simulink model "MPC(废稿)"  (R2023a)
settings: Solver=VariableStepAuto  StartTime=0.0  StopTime=50  RelTol=1e-3
settings Model: Creator=c  LastModifiedBy=c

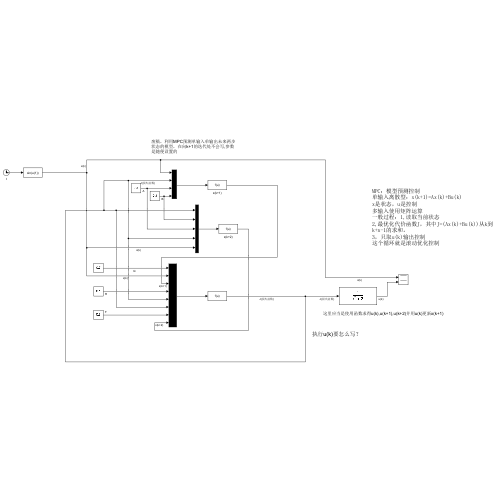
[thumbnail: Simulink's stored preview of the top-level diagram]
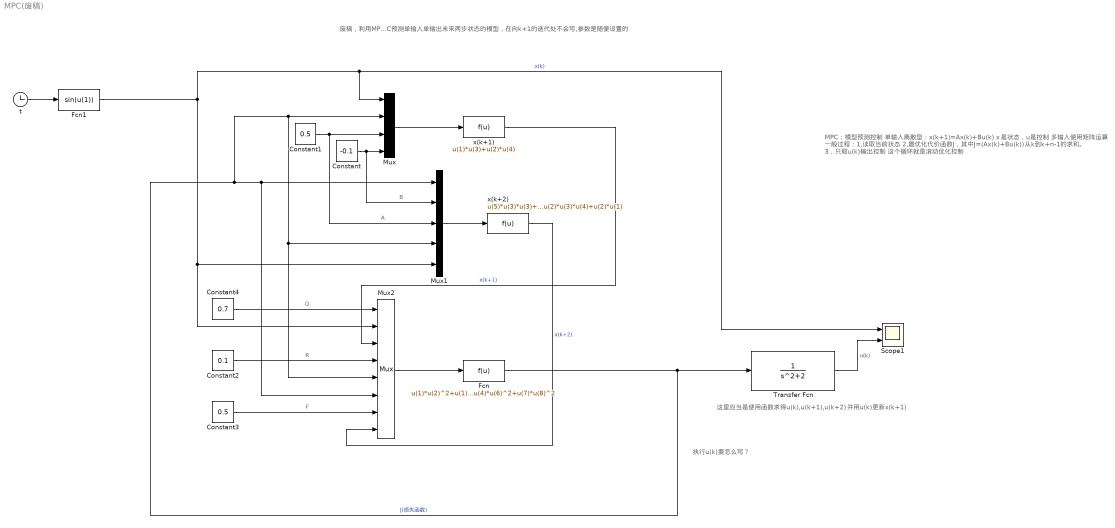
== system MPC(废稿) ==
  note: 废稿，利用MPC预测单输入单输出未来两步状态的模型，在向k+1的迭代处不会写,参数是随便设置的
  note: 这里应当是使用函数求得u(k),u(k+1),u(k+2)并用u(k)更新x(k+1)
  note: 执行u(k)要怎么写？
  note: MPC：模型预测控制
      | 单输入离散型：x(k+1)=Ax(k)+Bu(k)
      | x是状态，u是控制
      | 多输入使用矩阵运算
      | 一般过程：1,读取当前状态
      | 2,最优化代价函数J，其中J=(Ax(k)+Bu(k))从k到k+n-1的求和。
      | 3，只取u(k)输出控制
      | 这个循环就是滚动优化控制
  Constant : Constant  Value=-0.1
  Constant1 : Constant  Value=0.5
  Constant2 : Constant  Value=0.1
  Constant3 : Constant  Value=0.5
  Constant4 : Constant  Value=0.7
  Fcn : Fcn  Expr=u(1)*u(2)^2+u(1)*u(3)^2+u(4)*u(5)^2+u(4)*u(6)^2+u(7)*u(8)^2
  Fcn1 : Fcn  Expr=sin(u(1))
  Mux : Mux
  Mux1 : Mux  Inputs=5
  Mux2 : Mux  Inputs=8
  Scope1 : Scope  NumInputPorts=2
  Transfer Fcn : TransferFcn  Denominator=[1 0 2]
  t : Clock
  x(k+1) : Fcn  Expr=u(1)*u(3)+u(2)*u(4)
  x(k+2) : Fcn  Expr=u(5)*u(3)*u(3)+u(2)*u(3)*u(4)+u(2)*u(1)
  wires:
  Mux/1 -> x(k+1)/1
  Constant/1 -> Mux1/2, Mux/4  "B"
  Mux1/1 -> x(k+2)/1
  Constant1/1 -> Mux1/3, Mux/3  "A"
  Fcn/1 -> Transfer Fcn/1, Mux1/4, Mux2/5, Mux/2, Mux2/6, Mux1/1  "J(损失函数)"
  Mux2/1 -> Fcn/1
  Constant2/1 -> Mux2/4  "R"
  Constant3/1 -> Mux2/7  "F"
  x(k+2)/1 -> Mux2/8  "x(k+2)"
  Constant4/1 -> Mux2/1  "Q"
  x(k+1)/1 -> Mux2/3  "x(k+1)"
  Transfer Fcn/1 -> Scope1/2  "u(k)"
  Fcn1/1 -> Mux/1, Scope1/1, Mux2/2, Mux1/5  "x(k)"
  t/1 -> Fcn1/1
